simulink model "EulerPIDJoint_Copy"  (Simulink 7.6)
settings: Solver=ode3  StartTime=0.0  StopTime=8  FixedStep=Ts  RelTol=1e-3
InitFcn:
  | eval('Config');
  | eval('RobotCtlCfg');
values from neighbouring files (symbols this model uses):
  a2 = 0    [Config.m]    (also in CtrPlatformCfg.m)
  a3 = 0    [Config.m]    (also in CtrPlatformCfg.m)
  a4 = 0    [Config.m]    (also in CtrPlatformCfg.m)
  a5 = 90    [Config.m]    (also in CtrPlatformCfg.m)
  a6 = 0    [Config.m]    (also in CtrPlatformCfg.m)
  Cen_EU = Cen    [DynEulerTest.m]
  DH_EU = [266     300     0       0       1016     0      174 ... (first row only)    [DynEulerTest.m]
  freq = tvel/radius    (= 1)    [Config.m]    (also in CtrPlatformCfg.m)
  Ft_EU = [0;0;0;0;0;0]    [DynEulerTest.m]
  Gravity = 9.8    [Config.m]    (also in CtrPlatformCfg.m)
  Ie_EU = [Ie1;Ie2;Ie3;Ie4;Ie5;Ie6]    [DynEulerTest.m]
  in1 = [5.2954 -0.2565 -0.6366;-0.2565 4.7000 0.2830;-0.6366 0.2829 5.8635]    [Config.m]    (also in CtrPlatformCfg.m; DynEulerTest.m; EfDynCAD.m = [0.54  -0.01 0.23)
  in2 = [5.8840 0.0072 0.0135;0.0072 6.0178 -0.1907;0.0135 -0.1907 0.3374]    [Config.m]    (also in CtrPlatformCfg.m; DynEulerTest.m; EfDynCAD.m = (R_x*R_z)*in2*(R_x*R_z)')
  in3 = [1.8201 -0.2274 -0.3112;-0.2274 2.2537 -0.1441;-0.3112 -0.1441 1.9485]    [Config.m]    (also in CtrPlatformCfg.m; DynEulerTest.m; EfDynCAD.m = (R_x*R_z)*in3*(R_x*R_z)')
  in4 = [0.0607 -0.0922 0;-0.0922 1.4493 0;0 0 1.4620]    [Config.m]    (also in CtrPlatformCfg.m; DynEulerTest.m = [0.0607 -0.0922 0;-0.0922 1.4493 0;0 0,1.4620]; EfDynCAD.m = (R_y*Rz)*in4*(R_y*Rz)')
  in5 = [0.0191 0.0032 0;0.0032 0.0228 0;0 0 0.0291]    [Config.m]    (also in CtrPlatformCfg.m; DynEulerTest.m; EfDynCAD.m = (R_x*R_y)*in5*(R_x*R_y)')
  in6 = [0.0012 0 0;0 0.0007 0;0 0 0.0007]    [Config.m]    (also in CtrPlatformCfg.m; DynEulerTest.m; EfDynCAD.m = (R_y*Rz)*in6*(R_y*Rz)')
  init_Endx = gd_init(1,4)    [Config.m]    (also in CtrPlatformCfg.m)
  init_Endy = gd_init(2,4)    [Config.m]    (also in CtrPlatformCfg.m)
  init_Endz = gd_init(3,4)    [Config.m]    (also in CtrPlatformCfg.m)
  init_Rot = gd_init(1:3,1:3)    [Config.m]    (also in CtrPlatformCfg.m)
  L = [l1 l2 l3 l4 l5 l6 l7 l8 l9]    [Config.m]    (also in CtrPlatformCfg.m)
  ma1 = 170.31    [Config.m]    (also in CtrPlatformCfg.m; DynEulerTest.m; EfDynCAD.m = 77.75)
  ma2 = 63.74    [Config.m]    (also in CtrPlatformCfg.m; DynEulerTest.m; EfDynCAD.m = 32.31)
  ma3 = 98.98    [Config.m]    (also in CtrPlatformCfg.m; DynEulerTest.m; EfDynCAD.m = 18.61)
  ma4 = 24.46    [Config.m]    (also in CtrPlatformCfg.m; DynEulerTest.m; EfDynCAD.m = 15.65)
  ma5 = 5.24    [Config.m]    (also in CtrPlatformCfg.m; DynEulerTest.m; EfDynCAD.m = 3.32)
  ma6 = 0.6    [Config.m]    (also in CtrPlatformCfg.m; DynEulerTest.m; EfDynCAD.m)
  Ma_EU = Ma    [DynEulerTest.m]
  Rad2Line = Gear*EncRes/(2*pi)    [Config.m]    (also in CtrPlatformCfg.m)
  Ts = 1/FrHz    (= 0.00025)    [Config.m]    (also in CtrPlatformCfg.m)
  tvel = 120    [Config.m]    (also in CtrPlatformCfg.m)
undefined symbols (not defined in the file or in its folder): a1, DiscIntNeverNeededParam, jointAugKp, jointAugKv, PRBSGain, PRBSOffset, PRBSTimeLength, PulseFrq, PulseGain, RobotAxis, SineFrq, SineGain, V2T
libraries: simulink x58, mblibv1 x41, powerlib_extras x7
(part 3 of 5)

== system EulerPIDJoint_Copy/Display/GeneralForceDisplay/Jnt4 ==
  Enc : Inport
  Ref : Inport  Port=2
  Demux1 : Demux  Outputs=2
  Demux3 : Demux  Outputs=6
  Display : Subsystem
  Mux : Mux  Inputs=3
  Mux1 : Mux  Inputs=3
  Mux2 : Mux  Inputs=2
  Mux3 : Mux  Inputs=2
  Sign{1,3..4,6} (4 alike) : Gain
  Sign2 : Gain  Gain=-1
  Sign5 : Gain  Gain=-1
  wires:
  Mux3/1 -> Display/2(Ref_GeneralForce4)
  Mux2/1 -> Display/1(GeneralForce4)
  Sign5/1 -> Mux1/2
  Sign2/1 -> Mux/2
  Demux3/6 -> Sign6/1
  Demux3/5 -> Sign5/1
  Demux3/4 -> Sign4/1
  Demux3/3 -> Sign3/1
  Demux3/2 -> Sign2/1
  Demux3/1 -> Sign1/1
  Mux1/1 -> Mux3/2
  Mux/1 -> Mux3/1
  Ref/1 -> Demux3/1
  Enc/1 -> Demux1/1
  Sign1/1 -> Mux/3
  Sign3/1 -> Mux/1
  Sign4/1 -> Mux1/3
  Sign6/1 -> Mux1/1
  Demux1/1 -> Mux2/1
  Demux1/2 -> Mux2/2

== system EulerPIDJoint_Copy/Display/GeneralForceDisplay/Jnt5 ==
  Enc : Inport
  Ref : Inport  Port=2
  Demux1 : Demux  Outputs=2
  Demux3 : Demux  Outputs=6
  Display : Subsystem
  Mux : Mux  Inputs=3
  Mux1 : Mux  Inputs=3
  Mux2 : Mux  Inputs=2
  Mux3 : Mux  Inputs=2
  Sign{1,3..4,6} (4 alike) : Gain  Gain=-1
  Sign2 : Gain
  Sign5 : Gain
  wires:
  Enc/1 -> Demux1/1
  Ref/1 -> Demux3/1
  Mux/1 -> Mux3/1
  Mux1/1 -> Mux3/2
  Demux3/1 -> Sign1/1
  Demux3/2 -> Sign2/1
  Demux3/3 -> Sign3/1
  Demux3/4 -> Sign4/1
  Demux3/5 -> Sign5/1
  Demux3/6 -> Sign6/1
  Mux2/1 -> Display/1(GeneralForce5)
  Mux3/1 -> Display/2(Ref_GeneralForce5)
  Sign1/1 -> Mux/2
  Sign2/1 -> Mux/3
  Sign3/1 -> Mux/1
  Sign4/1 -> Mux1/2
  Sign5/1 -> Mux1/3
  Sign6/1 -> Mux1/1
  Demux1/1 -> Mux2/1
  Demux1/2 -> Mux2/2

== system EulerPIDJoint_Copy/Display/GeneralForceDisplay/Jnt6 ==
  Enc : Inport
  Ref : Inport  Port=2
  Demux1 : Demux  Outputs=2
  Demux3 : Demux  Outputs=6
  Display : Subsystem
  Mux : Mux  Inputs=3
  Mux1 : Mux  Inputs=3
  Mux2 : Mux  Inputs=2
  Mux3 : Mux  Inputs=2
  Sign{1,3..4,6} (4 alike) : Gain
  Sign2 : Gain  Gain=-1
  Sign5 : Gain  Gain=-1
  wires:
  Mux3/1 -> Display/2(Ref_GeneralForce6)
  Mux2/1 -> Display/1(GeneralForce6)
  Sign5/1 -> Mux1/2
  Sign2/1 -> Mux/2
  Demux3/6 -> Sign6/1
  Demux3/5 -> Sign5/1
  Demux3/4 -> Sign4/1
  Demux3/3 -> Sign3/1
  Demux3/2 -> Sign2/1
  Demux3/1 -> Sign1/1
  Mux1/1 -> Mux3/2
  Mux/1 -> Mux3/1
  Ref/1 -> Demux3/1
  Enc/1 -> Demux1/1
  Sign1/1 -> Mux/3
  Sign3/1 -> Mux/1
  Sign6/1 -> Mux1/1
  Sign4/1 -> Mux1/3
  Demux1/1 -> Mux2/1
  Demux1/2 -> Mux2/2

== system EulerPIDJoint_Copy/Display/GeneralVelDisplay/Jnt1 ==
  Enc : Inport
  Ref : Inport  Port=2
  Demux1 : Demux  Outputs=2
  Demux3 : Demux  Outputs=6
  Display : Subsystem
  Mux : Mux  Inputs=3
  Mux1 : Mux  Inputs=3
  Mux2 : Mux  Inputs=2
  Mux3 : Mux  Inputs=2
  Sign{1..6} (6 alike) : Gain
  wires:
  Enc/1 -> Demux1/1
  Ref/1 -> Demux3/1
  Mux/1 -> Mux3/1
  Mux1/1 -> Mux3/2
  Demux3/1 -> Sign1/1
  Demux3/2 -> Sign2/1
  Demux3/3 -> Sign3/1
  Demux3/4 -> Sign4/1
  Demux3/5 -> Sign5/1
  Demux3/6 -> Sign6/1
  Sign1/1 -> Mux/1
  Sign2/1 -> Mux/2
  Sign3/1 -> Mux/3
  Sign4/1 -> Mux1/1
  Sign5/1 -> Mux1/2
  Sign6/1 -> Mux1/3
  Demux1/1 -> Mux2/1
  Demux1/2 -> Mux2/2
  Mux2/1 -> Display/1(GeneralVel1)
  Mux3/1 -> Display/2(Ref_GeneralVel1)

== system EulerPIDJoint_Copy/Display/GeneralVelDisplay/Jnt2 ==
  Enc : Inport
  Ref : Inport  Port=2
  Demux1 : Demux  Outputs=2
  Demux3 : Demux  Outputs=6
  Display : Subsystem
  Mux : Mux  Inputs=3
  Mux1 : Mux  Inputs=3
  Mux2 : Mux  Inputs=2
  Mux3 : Mux  Inputs=2
  Sign{1..2,4..5} (4 alike) : Gain
  Sign3 : Gain  Gain=-1
  Sign6 : Gain  Gain=-1
  wires:
  Mux3/1 -> Display/2(Ref_GeneralVel2)
  Mux2/1 -> Display/1(GeneralVel2)
  Demux1/2 -> Mux2/2
  Demux1/1 -> Mux2/1
  Sign4/1 -> Mux1/1
  Sign1/1 -> Mux/1
  Demux3/6 -> Sign6/1
  Demux3/5 -> Sign5/1
  Demux3/4 -> Sign4/1
  Demux3/3 -> Sign3/1
  Demux3/2 -> Sign2/1
  Demux3/1 -> Sign1/1
  Mux1/1 -> Mux3/2
  Mux/1 -> Mux3/1
  Ref/1 -> Demux3/1
  Enc/1 -> Demux1/1
  Sign3/1 -> Mux/2
  Sign2/1 -> Mux/3
  Sign6/1 -> Mux1/2
  Sign5/1 -> Mux1/3

== system EulerPIDJoint_Copy/Display/GeneralVelDisplay/Jnt3 ==
  Enc : Inport
  Ref : Inport  Port=2
  Demux1 : Demux  Outputs=2
  Demux3 : Demux  Outputs=6
  Display : Subsystem
  Mux : Mux  Inputs=3
  Mux1 : Mux  Inputs=3
  Mux2 : Mux  Inputs=2
  Mux3 : Mux  Inputs=2
  Sign{1..6} (6 alike) : Gain
  wires:
  Enc/1 -> Demux1/1
  Ref/1 -> Demux3/1
  Mux/1 -> Mux3/1
  Mux1/1 -> Mux3/2
  Demux3/1 -> Sign1/1
  Demux3/2 -> Sign2/1
  Demux3/3 -> Sign3/1
  Demux3/4 -> Sign4/1
  Demux3/5 -> Sign5/1
  Demux3/6 -> Sign6/1
  Demux1/1 -> Mux2/1
  Demux1/2 -> Mux2/2
  Mux2/1 -> Display/1(GeneralVel3)
  Mux3/1 -> Display/2(Ref_GeneralVel3)
  Sign1/1 -> Mux/2
  Sign2/1 -> Mux/3
  Sign3/1 -> Mux/1
  Sign4/1 -> Mux1/2
  Sign6/1 -> Mux1/1
  Sign5/1 -> Mux1/3

== system EulerPIDJoint_Copy/Display/GeneralVelDisplay/Jnt4 ==
  Enc : Inport
  Ref : Inport  Port=2
  Demux1 : Demux  Outputs=2
  Demux3 : Demux  Outputs=6
  Display : Subsystem
  Mux : Mux  Inputs=3
  Mux1 : Mux  Inputs=3
  Mux2 : Mux  Inputs=2
  Mux3 : Mux  Inputs=2
  Sign{1,3..4,6} (4 alike) : Gain
  Sign2 : Gain  Gain=-1
  Sign5 : Gain  Gain=-1
  wires:
  Mux3/1 -> Display/2(Ref_GeneralVel4)
  Mux2/1 -> Display/1(GeneralVel4)
  Sign5/1 -> Mux1/2
  Sign2/1 -> Mux/2
  Demux3/6 -> Sign6/1
  Demux3/5 -> Sign5/1
  Demux3/4 -> Sign4/1
  Demux3/3 -> Sign3/1
  Demux3/2 -> Sign2/1
  Demux3/1 -> Sign1/1
  Mux1/1 -> Mux3/2
  Mux/1 -> Mux3/1
  Ref/1 -> Demux3/1
  Enc/1 -> Demux1/1
  Sign1/1 -> Mux/3
  Sign3/1 -> Mux/1
  Sign4/1 -> Mux1/3
  Sign6/1 -> Mux1/1
  Demux1/1 -> Mux2/1
  Demux1/2 -> Mux2/2

== system EulerPIDJoint_Copy/Display/GeneralVelDisplay/Jnt5 ==
  Enc : Inport
  Ref : Inport  Port=2
  Demux1 : Demux  Outputs=2
  Demux3 : Demux  Outputs=6
  Display : Subsystem
  Mux : Mux  Inputs=3
  Mux1 : Mux  Inputs=3
  Mux2 : Mux  Inputs=2
  Mux3 : Mux  Inputs=2
  Sign{1,3..4,6} (4 alike) : Gain  Gain=-1
  Sign2 : Gain
  Sign5 : Gain
  wires:
  Enc/1 -> Demux1/1
  Ref/1 -> Demux3/1
  Mux/1 -> Mux3/1
  Mux1/1 -> Mux3/2
  Demux3/1 -> Sign1/1
  Demux3/2 -> Sign2/1
  Demux3/3 -> Sign3/1
  Demux3/4 -> Sign4/1
  Demux3/5 -> Sign5/1
  Demux3/6 -> Sign6/1
  Mux2/1 -> Display/1(GeneralVel5)
  Mux3/1 -> Display/2(Ref_GeneralVel5)
  Sign1/1 -> Mux/2
  Sign2/1 -> Mux/3
  Sign3/1 -> Mux/1
  Sign4/1 -> Mux1/2
  Sign5/1 -> Mux1/3
  Sign6/1 -> Mux1/1
  Demux1/1 -> Mux2/1
  Demux1/2 -> Mux2/2

== system EulerPIDJoint_Copy/Display/GeneralVelDisplay/Jnt6 ==
  Enc : Inport
  Ref : Inport  Port=2
  Demux1 : Demux  Outputs=2
  Demux3 : Demux  Outputs=6
  Display : Subsystem
  Mux : Mux  Inputs=3
  Mux1 : Mux  Inputs=3
  Mux2 : Mux  Inputs=2
  Mux3 : Mux  Inputs=2
  Sign{1,3..4,6} (4 alike) : Gain
  Sign2 : Gain  Gain=-1
  Sign5 : Gain  Gain=-1
  wires:
  Mux3/1 -> Display/2(Ref_GeneralVel6)
  Mux2/1 -> Display/1(GeneralVel6)
  Sign5/1 -> Mux1/2
  Sign2/1 -> Mux/2
  Demux3/6 -> Sign6/1
  Demux3/5 -> Sign5/1
  Demux3/4 -> Sign4/1
  Demux3/3 -> Sign3/1
  Demux3/2 -> Sign2/1
  Demux3/1 -> Sign1/1
  Mux1/1 -> Mux3/2
  Mux/1 -> Mux3/1
  Ref/1 -> Demux3/1
  Enc/1 -> Demux1/1
  Sign1/1 -> Mux/3
  Sign3/1 -> Mux/1
  Sign6/1 -> Mux1/1
  Sign4/1 -> Mux1/3
  Demux1/1 -> Mux2/1
  Demux1/2 -> Mux2/2

== system EulerPIDJoint_Copy/Display/JntVelAccDisplay/Joint1 ==
  JVA1 : Inport
  Ref_JVA1 : Inport  Port=2
  Acceleration : Scope
      settings: SaveName=ScopeData2
  Angle : Scope
      settings: TimeRange=10  YMin=-3e-017  YMax=4e-017
  Demux : Demux  Outputs=3
  Demux1 : Demux  Outputs=3
  "Encoder " : ToWorkspace  VariableName=EncJVAJ1  SampleTime=-1  SaveFormat=Structure
  Err1 : Scope
      settings: SaveName=ScopeData6
  Err2 : Scope
      settings: SaveName=ScopeData7
  Err3 : Scope
      settings: SaveName=ScopeData8
  Mux : Mux  Inputs=2
  Mux1 : Mux  Inputs=2
  Mux2 : Mux  Inputs=2
  "Ref " : ToWorkspace  VariableName=RefJVAJ1  SampleTime=-1  SaveFormat=Structure
  Sum : Sum  Inputs=+|-
  Sum1 : Sum  Inputs=+|-
  Sum2 : Sum  Inputs=+|-
  "Velocity " : Scope
  wires:
  Ref_JVA1/1 -> "Ref "/1, Demux1/1
  JVA1/1 -> "Encoder "/1, Demux/1
  Sum2/1 -> Err3/1
  Sum1/1 -> Err2/1
  Sum/1 -> Err1/1
  Demux/1 -> Sum/1, Mux/1
  Demux1/1 -> Sum/2, Mux/2
  Demux/2 -> Sum1/1, Mux1/1
  Demux1/2 -> Sum1/2, Mux1/2
  Demux/3 -> Sum2/1, Mux2/1
  Demux1/3 -> Sum2/2, Mux2/2
  Mux/1 -> Angle/1
  Mux1/1 -> "Velocity "/1
  Mux2/1 -> Acceleration/1

== system EulerPIDJoint_Copy/Display/JntVelAccDisplay/Joint2 ==
  JVA2 : Inport
  Ref_JVA2 : Inport  Port=2
  Acceleration : Scope
      settings: SaveName=ScopeData2
  Angle : Scope
      settings: TimeRange=10  YMin=-3e-017  YMax=4e-017
  Demux : Demux  Outputs=3
  Demux1 : Demux  Outputs=3
  "Encoder " : ToWorkspace  VariableName=EncJVAJ2  SampleTime=-1  SaveFormat=Structure
  Err1 : Scope
      settings: SaveName=ScopeData6
  Err2 : Scope
      settings: SaveName=ScopeData7
  Err3 : Scope
      settings: SaveName=ScopeData8
  Mux : Mux  Inputs=2
  Mux1 : Mux  Inputs=2
  Mux2 : Mux  Inputs=2
  "Ref " : ToWorkspace  VariableName=RefJVAJ2  SampleTime=-1  SaveFormat=Structure
  Sum : Sum  Inputs=+|-
  Sum1 : Sum  Inputs=+|-
  Sum2 : Sum  Inputs=+|-
  "Velocity " : Scope
  wires:
  Mux2/1 -> Acceleration/1
  Mux1/1 -> "Velocity "/1
  Mux/1 -> Angle/1
  Demux1/3 -> Mux2/2, Sum2/2
  Demux/3 -> Mux2/1, Sum2/1
  Demux1/2 -> Mux1/2, Sum1/2
  Demux/2 -> Mux1/1, Sum1/1
  Demux1/1 -> Mux/2, Sum/2
  Demux/1 -> Mux/1, Sum/1
  Sum/1 -> Err1/1
  Sum1/1 -> Err2/1
  Sum2/1 -> Err3/1
  JVA2/1 -> Demux/1, "Encoder "/1
  Ref_JVA2/1 -> Demux1/1, "Ref "/1

== system EulerPIDJoint_Copy/Display/JntVelAccDisplay/Joint3 ==
  JVA3 : Inport
  Ref_JVA3 : Inport  Port=2
  Acceleration : Scope
      settings: SaveName=ScopeData2
  Angle : Scope
      settings: TimeRange=10  YMin=-3e-017  YMax=4e-017
  Demux : Demux  Outputs=3
  Demux1 : Demux  Outputs=3
  "Encoder " : ToWorkspace  VariableName=EncJVAJ3  SampleTime=-1  SaveFormat=Structure
  Err1 : Scope
      settings: SaveName=ScopeData6
  Err2 : Scope
      settings: SaveName=ScopeData7
  Err3 : Scope
      settings: SaveName=ScopeData8
  Mux : Mux  Inputs=2
  Mux1 : Mux  Inputs=2
  Mux2 : Mux  Inputs=2
  "Ref " : ToWorkspace  VariableName=RefJVAJ3  SampleTime=-1  SaveFormat=Structure
  Sum : Sum  Inputs=+|-
  Sum1 : Sum  Inputs=+|-
  Sum2 : Sum  Inputs=+|-
  "Velocity " : Scope
  wires:
  Ref_JVA3/1 -> "Ref "/1, Demux1/1
  JVA3/1 -> "Encoder "/1, Demux/1
  Sum2/1 -> Err3/1
  Sum1/1 -> Err2/1
  Sum/1 -> Err1/1
  Demux/1 -> Sum/1, Mux/1
  Demux1/1 -> Sum/2, Mux/2
  Demux/2 -> Sum1/1, Mux1/1
  Demux1/2 -> Sum1/2, Mux1/2
  Demux/3 -> Sum2/1, Mux2/1
  Demux1/3 -> Sum2/2, Mux2/2
  Mux/1 -> Angle/1
  Mux1/1 -> "Velocity "/1
  Mux2/1 -> Acceleration/1

== system EulerPIDJoint_Copy/Display/JntVelAccDisplay/Joint4 ==
  JVA4 : Inport
  Ref_JVA4 : Inport  Port=2
  Acceleration : Scope
      settings: SaveName=ScopeData2
  Angle : Scope
      settings: TimeRange=10  YMin=-3e-017  YMax=4e-017
  Demux : Demux  Outputs=3
  Demux1 : Demux  Outputs=3
  "Encoder " : ToWorkspace  VariableName=EncJVAJ4  SampleTime=-1  SaveFormat=Structure
  Err1 : Scope
      settings: SaveName=ScopeData6
  Err2 : Scope
      settings: SaveName=ScopeData7
  Err3 : Scope
      settings: SaveName=ScopeData8
  Mux : Mux  Inputs=2
  Mux1 : Mux  Inputs=2
  Mux2 : Mux  Inputs=2
  "Ref " : ToWorkspace  VariableName=RefJVAJ4  SampleTime=-1  SaveFormat=Structure
  Sum : Sum  Inputs=+|-
  Sum1 : Sum  Inputs=+|-
  Sum2 : Sum  Inputs=+|-
  "Velocity " : Scope
  wires:
  Mux2/1 -> Acceleration/1
  Mux1/1 -> "Velocity "/1
  Mux/1 -> Angle/1
  Demux1/3 -> Mux2/2, Sum2/2
  Demux/3 -> Mux2/1, Sum2/1
  Demux1/2 -> Mux1/2, Sum1/2
  Demux/2 -> Mux1/1, Sum1/1
  Demux1/1 -> Mux/2, Sum/2
  Demux/1 -> Mux/1, Sum/1
  Sum/1 -> Err1/1
  Sum1/1 -> Err2/1
  Sum2/1 -> Err3/1
  JVA4/1 -> Demux/1, "Encoder "/1
  Ref_JVA4/1 -> Demux1/1, "Ref "/1

== system EulerPIDJoint_Copy/Display/JntVelAccDisplay/Joint5 ==
  JVA5 : Inport
  Ref_JVA5 : Inport  Port=2
  Acceleration : Scope
      settings: SaveName=ScopeData2
  Angle : Scope
      settings: TimeRange=10  YMin=-3e-017  YMax=4e-017
  Demux : Demux  Outputs=3
  Demux1 : Demux  Outputs=3
  "Encoder " : ToWorkspace  VariableName=EncJVAJ5  SampleTime=-1  SaveFormat=Structure
  Err1 : Scope
      settings: SaveName=ScopeData6
  Err2 : Scope
      settings: SaveName=ScopeData7
  Err3 : Scope
      settings: SaveName=ScopeData8
  Mux : Mux  Inputs=2
  Mux1 : Mux  Inputs=2
  Mux2 : Mux  Inputs=2
  "Ref " : ToWorkspace  VariableName=RefJVAJ5  SampleTime=-1  SaveFormat=Structure
  Sum : Sum  Inputs=+|-
  Sum1 : Sum  Inputs=+|-
  Sum2 : Sum  Inputs=+|-
  "Velocity " : Scope
  wires:
  Ref_JVA5/1 -> "Ref "/1, Demux1/1
  JVA5/1 -> "Encoder "/1, Demux/1
  Sum2/1 -> Err3/1
  Sum1/1 -> Err2/1
  Sum/1 -> Err1/1
  Demux/1 -> Sum/1, Mux/1
  Demux1/1 -> Sum/2, Mux/2
  Demux/2 -> Sum1/1, Mux1/1
  Demux1/2 -> Sum1/2, Mux1/2
  Demux/3 -> Sum2/1, Mux2/1
  Demux1/3 -> Sum2/2, Mux2/2
  Mux/1 -> Angle/1
  Mux1/1 -> "Velocity "/1
  Mux2/1 -> Acceleration/1

== system EulerPIDJoint_Copy/Display/JntVelAccDisplay/Joint6 ==
  JVA6 : Inport
  Ref_JVA6 : Inport  Port=2
  Acceleration : Scope
      settings: SaveName=ScopeData2
  Angle : Scope
      settings: TimeRange=10  YMin=-3e-017  YMax=4e-017
  Demux : Demux  Outputs=3
  Demux1 : Demux  Outputs=3
  "Encoder " : ToWorkspace  VariableName=EncJVAJ6  SampleTime=-1  SaveFormat=Structure
  Err1 : Scope
      settings: SaveName=ScopeData6
  Err2 : Scope
      settings: SaveName=ScopeData7
  Err3 : Scope
      settings: SaveName=ScopeData8
  Mux : Mux  Inputs=2
  Mux1 : Mux  Inputs=2
  Mux2 : Mux  Inputs=2
  "Ref " : ToWorkspace  VariableName=RefJVAJ6  SampleTime=-1  SaveFormat=Structure
  Sum : Sum  Inputs=+|-
  Sum1 : Sum  Inputs=+|-
  Sum2 : Sum  Inputs=+|-
  "Velocity " : Scope
  wires:
  Mux2/1 -> Acceleration/1
  Mux1/1 -> "Velocity "/1
  Mux/1 -> Angle/1
  Demux1/3 -> Mux2/2, Sum2/2
  Demux/3 -> Mux2/1, Sum2/1
  Demux1/2 -> Mux1/2, Sum1/2
  Demux/2 -> Mux1/1, Sum1/1
  Demux1/1 -> Mux/2, Sum/2
  Demux/1 -> Mux/1, Sum/1
  Sum/1 -> Err1/1
  Sum1/1 -> Err2/1
  Sum2/1 -> Err3/1
  JVA6/1 -> Demux/1, "Encoder "/1
  Ref_JVA6/1 -> Demux1/1, "Ref "/1

== system EulerPIDJoint_Copy/Trajectory Generator/Circle in Descartes Space/EndVelocity ==
  Constant : Constant  Value=-1  SampleTime=Ts
  End_Vx : Sin  Amplitude=-tvel  Frequency=freq  SampleTime=Ts
  End_Vy : Sin  Frequency=freq  Phase=pi/2  SampleTime=Ts
  End_Vz : Constant  Value=0  SampleTime=Ts
  Gain : Gain  Gain=tvel
  Integer Delay : simulink/Discrete/Integer Delay  NumDelays=1/Ts  vinit=0.0  samptime=-1
  Integer Delay1 : simulink/Discrete/Integer Delay  NumDelays=1/Ts  vinit=0.0  samptime=-1
  Ramp : simulink/Sources/Ramp  SystemSampleTime=-1  slope=1  start=0  X0=0
  Ramp1 : simulink/Sources/Ramp  SystemSampleTime=-1  slope=-1  start=1  X0=0
  Sum : Sum  Inputs=|++
  Sum1 : Sum  Inputs=++|  SampleTime=Ts
  Sum2 : Sum  Inputs=++|
  EndVx : Outport
  EndVy : Outport  Port=2
  EndVz : Outport  Port=3
  wires:
  End_Vy/1 -> Sum2/1
  Ramp/1 -> Sum/1
  Ramp1/1 -> Sum/2
  Integer Delay1/1 -> Sum1/1
  Sum2/1 -> Integer Delay1/1
  Constant/1 -> Sum2/2
  Sum/1 -> Sum1/2
  Sum1/1 -> Gain/1
  End_Vx/1 -> Integer Delay/1
  End_Vz/1 -> EndVx/1
  Gain/1 -> EndVy/1
  Integer Delay/1 -> EndVz/1

== system EulerPIDJoint_Copy/Trajectory Generator/Circle in Descartes Space/Re-group  ==
  JJVVAA : Inport
  Demux2 : Demux  Outputs=18
  Mux{,1..2,4..6} (6 alike) : Mux  Inputs=3
  Mux3 : Mux  Inputs=6
  JVAJVA : Outport
  wires:
  JJVVAA/1 -> Demux2/1
  Mux3/1 -> JVAJVA/1
  Mux/1 -> Mux3/1
  Mux1/1 -> Mux3/2
  Mux2/1 -> Mux3/3
  Mux4/1 -> Mux3/4
  Mux5/1 -> Mux3/5
  Mux6/1 -> Mux3/6
  Demux2/1 -> Mux/1
  Demux2/2 -> Mux1/1
  Demux2/3 -> Mux2/1
  Demux2/4 -> Mux4/1
  Demux2/5 -> Mux5/1
  Demux2/6 -> Mux6/1
  Demux2/7 -> Mux/2
  Demux2/8 -> Mux1/2
  Demux2/9 -> Mux2/2
  Demux2/10 -> Mux4/2
  Demux2/11 -> Mux5/2
  Demux2/12 -> Mux6/2
  Demux2/13 -> Mux/3
  Demux2/14 -> Mux1/3
  Demux2/15 -> Mux2/3
  Demux2/16 -> Mux4/3
  Demux2/17 -> Mux5/3
  Demux2/18 -> Mux6/3

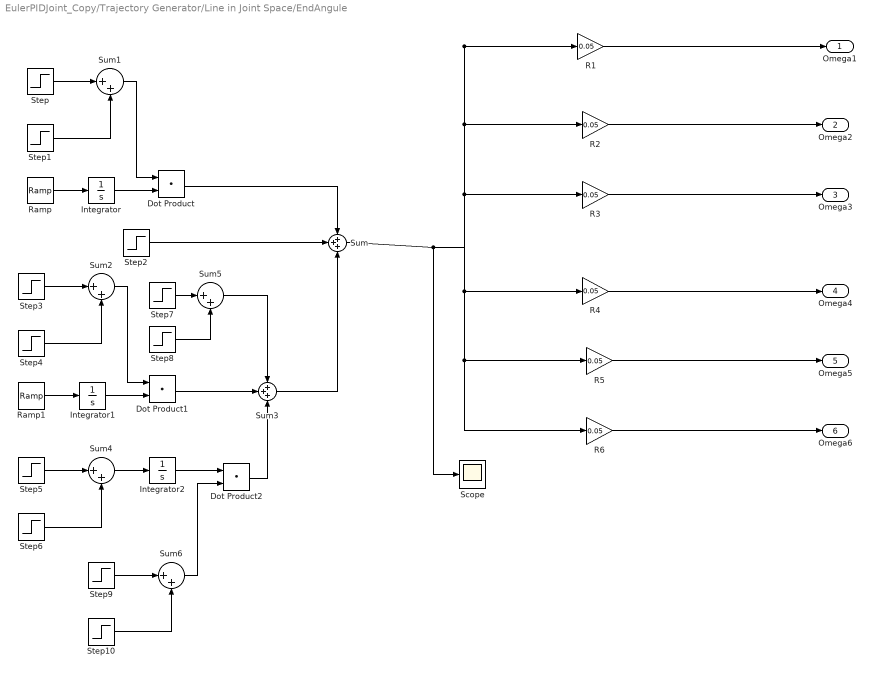
== system EulerPIDJoint_Copy/Trajectory Generator/Line in Joint Space/EndAngule ==
  Dot Product : DotProduct  InputSameDT=on  OutDataTypeStr=Inherit: Inherit via internal rule
  Dot Product1 : DotProduct  InputSameDT=on  OutDataTypeStr=Inherit: Inherit via internal rule
  Dot Product2 : DotProduct  InputSameDT=on  OutDataTypeStr=Inherit: Inherit via internal rule
  Integrator : Integrator
  Integrator1 : Integrator
  Integrator2 : Integrator
  R{1..6} (6 alike) : Gain  Gain=0.05
  Ramp : simulink/Sources/Ramp  SystemSampleTime=-1  slope=1  start=0  X0=0
  Ramp1 : simulink/Sources/Ramp  SystemSampleTime=-1  slope=-1  start=0  X0=0
  Scope : Scope
      settings: SaveName=ScopeData21
  Step : Step  After=-1  SampleTime=0
  Step1 : Step  Time=0  SampleTime=0
  Step10 : Step  SampleTime=0
  Step2 : Step  Time=2  SampleTime=0
  Step3 : Step  Time=2  After=-1  SampleTime=0
  Step4 : Step  SampleTime=0
  Step5 : Step  Time=2  After=-2  SampleTime=0
  Step6 : Step  After=2  SampleTime=0
  Step7 : Step  Time=2  After=-1  SampleTime=0
  Step8 : Step  SampleTime=0
  Step9 : Step  Time=2  After=-1  SampleTime=0
  Sum : Sum  Inputs=+++
  Sum{1..2,4..6} (5 alike) : Sum  Inputs=|++
  Sum3 : Sum  Inputs=+++
  Omega1 : Outport
  Omega2 : Outport  Port=2
  Omega3 : Outport  Port=3
  Omega4 : Outport  Port=4
  Omega5 : Outport  Port=5
  Omega6 : Outport  Port=6
  wires:
  R4/1 -> Omega4/1
  R6/1 -> Omega6/1
  R5/1 -> Omega5/1
  R3/1 -> Omega3/1
  R2/1 -> Omega2/1
  Ramp/1 -> Integrator/1
  R1/1 -> Omega1/1
  Sum/1 -> R1/1, R2/1, R3/1, R4/1, R5/1, R6/1, Scope/1
  Integrator/1 -> Dot Product/2
  Step/1 -> Sum1/1
  Sum1/1 -> Dot Product/1
  Step1/1 -> Sum1/2
  Dot Product/1 -> Sum/1
  Step2/1 -> Sum/2
  Ramp1/1 -> Integrator1/1
  Integrator1/1 -> Dot Product1/2
  Step3/1 -> Sum2/1
  Sum2/1 -> Dot Product1/1
  Step4/1 -> Sum2/2
  Sum3/1 -> Sum/3
  Step5/1 -> Sum4/1
  Step6/1 -> Sum4/2
  Sum4/1 -> Integrator2/1
  Dot Product1/1 -> Sum3/2
  Step7/1 -> Sum5/1
  Step8/1 -> Sum5/2
  Sum5/1 -> Sum3/1
  Step9/1 -> Sum6/1
  Step10/1 -> Sum6/2
  Integrator2/1 -> Dot Product2/1
  Sum6/1 -> Dot Product2/2
  Dot Product2/1 -> Sum3/3

== system EulerPIDJoint_Copy/Trajectory Generator/Line in Joint Space/Re-group  ==
  JJVVAA : Inport
  Demux2 : Demux  Outputs=18
  Mux{,1..2,4..6} (6 alike) : Mux  Inputs=3
  Mux3 : Mux  Inputs=6
  JVAJVA : Outport
  wires:
  JJVVAA/1 -> Demux2/1
  Mux3/1 -> JVAJVA/1
  Mux/1 -> Mux3/1
  Mux1/1 -> Mux3/2
  Mux2/1 -> Mux3/3
  Mux4/1 -> Mux3/4
  Mux5/1 -> Mux3/5
  Mux6/1 -> Mux3/6
  Demux2/1 -> Mux/1
  Demux2/2 -> Mux1/1
  Demux2/3 -> Mux2/1
  Demux2/4 -> Mux4/1
  Demux2/5 -> Mux5/1
  Demux2/6 -> Mux6/1
  Demux2/7 -> Mux/2
  Demux2/8 -> Mux1/2
  Demux2/9 -> Mux2/2
  Demux2/10 -> Mux4/2
  Demux2/11 -> Mux5/2
  Demux2/12 -> Mux6/2
  Demux2/13 -> Mux/3
  Demux2/14 -> Mux1/3
  Demux2/15 -> Mux2/3
  Demux2/16 -> Mux4/3
  Demux2/17 -> Mux5/3
  Demux2/18 -> Mux6/3

== system EulerPIDJoint_Copy/Trajectory Generator/Still/EndVelocity ==
  Constant : Constant  Value=0
  Constant1 : Constant  Value=0
  Constant2 : Constant  Value=0
  EndVx : Outport
  EndVy : Outport  Port=2
  EndVz : Outport  Port=3
  wires:
  Constant/1 -> EndVx/1
  Constant1/1 -> EndVy/1
  Constant2/1 -> EndVz/1

== system EulerPIDJoint_Copy/Trajectory Generator/Still/Re-group  ==
  JJVVAA : Inport
  Demux2 : Demux  Outputs=18
  Mux{,1..2,4..6} (6 alike) : Mux  Inputs=3
  Mux3 : Mux  Inputs=6
  JVAJVA : Outport
  wires:
  Demux2/18 -> Mux6/3
  Demux2/17 -> Mux5/3
  Demux2/16 -> Mux4/3
  Demux2/15 -> Mux2/3
  Demux2/14 -> Mux1/3
  Demux2/13 -> Mux/3
  Demux2/12 -> Mux6/2
  Demux2/11 -> Mux5/2
  Demux2/10 -> Mux4/2
  Demux2/9 -> Mux2/2
  Demux2/8 -> Mux1/2
  Demux2/7 -> Mux/2
  Demux2/6 -> Mux6/1
  Demux2/5 -> Mux5/1
  Demux2/4 -> Mux4/1
  Demux2/3 -> Mux2/1
  Demux2/2 -> Mux1/1
  Demux2/1 -> Mux/1
  Mux6/1 -> Mux3/6
  Mux5/1 -> Mux3/5
  Mux4/1 -> Mux3/4
  Mux2/1 -> Mux3/3
  Mux1/1 -> Mux3/2
  Mux/1 -> Mux3/1
  Mux3/1 -> JVAJVA/1
  JJVVAA/1 -> Demux2/1

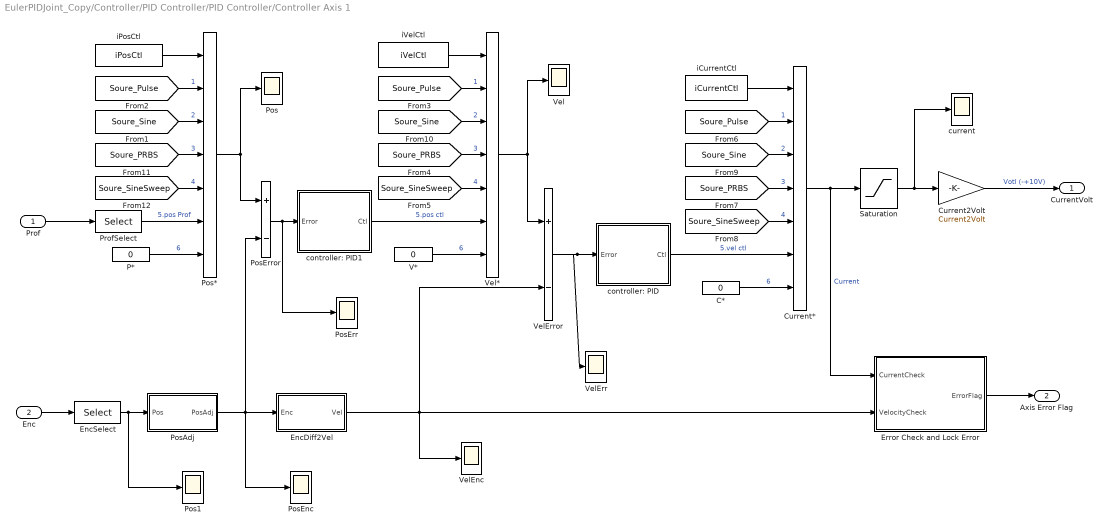
== system EulerPIDJoint_Copy/Controller/PID Controller/PID Controller/Controller Axis 1 ==
  Prof : Inport
  Enc : Inport  Port=2
  C* : Constant  Value=0  SampleTime=Ts
  Current* : MultiPortSwitch  Inputs=6  zeroidx=off
  Current2Volt : Gain  Gain=Current2Volt
  EncDiff2Vel : Subsystem
  "EncSelect " : Selector  InputPortWidth=6  IndexOptions=Index vector (dialog)  Indices=AxisNO  OutputSizes=1
  Error Check and Lock Error : Subsystem
  P* : Constant  Value=0  SampleTime=Ts
  Pos : Scope
      settings: TimeRange=1.4  YMin=-1  YMax=1  SaveName=ScopeData2
  Pos* : MultiPortSwitch  Inputs=6  zeroidx=off
  Pos1 : Scope
      settings: TimeRange=10  YMin=-1  YMax=1  SaveName=ScopeData43
  PosAdj : Subsystem
  PosEnc : Scope
      settings: TimeRange=10  YMin=-1  YMax=1  SaveName=ScopeData44
  PosErr : Scope
      settings: TimeRange=10  YMin=-1  YMax=1  SaveName=ScopeData42
  PosError : Sum  Inputs=+-
  ProfSelect : Selector  InputPortWidth=6  IndexOptions=Index vector (dialog)  Indices=AxisNO  OutputSizes=1
  Saturation : Saturate  UpperLimit=VLLimit %A  LowerLimit=-VLLimit %A  SampleTime=Ts
      settings: AttributesFormatString=%<UpperLimit>\n%<LowerLimit>
  V* : Constant  Value=0  SampleTime=Ts
  Vel : Scope
      settings: TimeRange=10  YMin=-1  YMax=1  SaveName=ScopeData5
  Vel* : MultiPortSwitch  Inputs=6  zeroidx=off
  VelEnc : Scope
      settings: TimeRange=10  YMin=-1  YMax=1  SaveName=ScopeData45
  VelErr : Scope
      settings: TimeRange=10  YMin=-1  YMax=1  SaveName=ScopeData46
  VelError : Sum  Inputs=+-
  controller: PID : Subsystem  mask{Kp=VLKp, Ki=VLKi, Kd=0, LimitSet=VLLimit, Ts=Ts}
      mask prompts: LimitSet "Limit of Int"; Ts "Sample Time"
  controller: PID1 : Subsystem  mask{Kp=PLKp, Ki=0, Kd=0, LimitSet=PLLimit, Ts=Ts}
      mask prompts: LimitSet "Limit of Int"; Ts "Sample Time"
  current : Scope
      settings: TimeRange=12  YMin=-9  YMax=9  SaveName=ScopeData3
  iCurrentCtl : Constant  Value=iCurrentCtl  SampleTime=Ts
  iPosCtl : Constant  Value=iPosCtl  SampleTime=Ts
  iVelCtl : Constant  Value=iVelCtl  SampleTime=Ts
  CurrentVolt : Outport
  Axis Error Flag : Outport  Port=2
  wires:
  Error Check and Lock Error/1(ErrorFlag) -> Axis Error Flag/1
  Saturation/1 -> current/1, Current2Volt/1
  Current*/1 -> Error Check and Lock Error/1(CurrentCheck), Saturation/1  "Current"
  PosError/1 -> controller: PID1/1(Error), PosErr/1
  iCurrentCtl/1 -> Current*/1
  iVelCtl/1 -> Vel*/1
  VelError/1 -> controller: PID/1(Error), VelErr/1
  controller: PID1/1(Ctl) -> Vel*/6  "5.pos ctl"
  PosAdj/1(PosAdj) -> EncDiff2Vel/1(Enc), PosEnc/1, PosError/2
  EncDiff2Vel/1(Vel) -> Error Check and Lock Error/2(VelocityCheck), VelEnc/1, VelError/2
  Prof/1 -> ProfSelect/1
  Enc/1 -> "EncSelect "/1
  "EncSelect "/1 -> PosAdj/1(Pos), Pos1/1
  [Soure_Pulse] -> Current*/2  "1"
  [Soure_Sine] -> Current*/3  "2"
  [Soure_PRBS] -> Current*/4  "3"
  [Soure_SineSweep] -> Current*/5  "4"
  controller: PID/1(Ctl) -> Current*/6  "5.vel ctl"
  C*/1 -> Current*/7  "6"
  [Soure_Pulse] -> Vel*/2  "1"
  [Soure_Sine] -> Vel*/3  "2"
  [Soure_PRBS] -> Vel*/4  "3"
  [Soure_SineSweep] -> Vel*/5  "4"
  V*/1 -> Vel*/7  "6"
  Vel*/1 -> Vel/1, VelError/1
  iPosCtl/1 -> Pos*/1
  ProfSelect/1 -> Pos*/6  "5.pos Prof"
  [Soure_Pulse] -> Pos*/2  "1"
  [Soure_Sine] -> Pos*/3  "2"
  [Soure_PRBS] -> Pos*/4  "3"
  [Soure_SineSweep] -> Pos*/5  "4"
  P*/1 -> Pos*/7  "6"
  Pos*/1 -> PosError/1, Pos/1
  Current2Volt/1 -> CurrentVolt/1  "Votl (-+10V)"

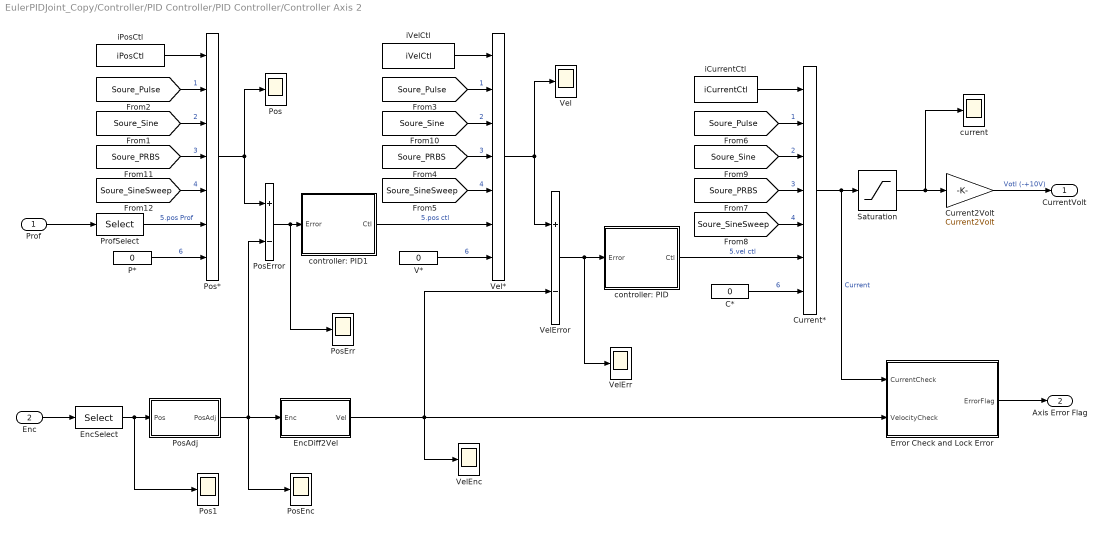
== system EulerPIDJoint_Copy/Controller/PID Controller/PID Controller/Controller Axis 2 ==
  Prof : Inport
  Enc : Inport  Port=2
  C* : Constant  Value=0  SampleTime=Ts
  Current* : MultiPortSwitch  Inputs=6  zeroidx=off
  Current2Volt : Gain  Gain=Current2Volt
  EncDiff2Vel : Subsystem
  "EncSelect " : Selector  InputPortWidth=6  IndexOptions=Index vector (dialog)  Indices=AxisNO  OutputSizes=1
  Error Check and Lock Error : Subsystem
  P* : Constant  Value=0  SampleTime=Ts
  Pos : Scope
      settings: TimeRange=1.4  YMin=-1  YMax=1  SaveName=ScopeData2
  Pos* : MultiPortSwitch  Inputs=6  zeroidx=off
  Pos1 : Scope
      settings: TimeRange=10  YMin=-1  YMax=1  SaveName=ScopeData35
  PosAdj : Subsystem
  PosEnc : Scope
      settings: TimeRange=10  YMin=-1  YMax=1  SaveName=ScopeData39
  PosErr : Scope
      settings: TimeRange=10  YMin=-1  YMax=1  SaveName=ScopeData34
  PosError : Sum  Inputs=+-
  ProfSelect : Selector  InputPortWidth=6  IndexOptions=Index vector (dialog)  Indices=AxisNO  OutputSizes=1
  Saturation : Saturate  UpperLimit=VLLimit %A  LowerLimit=-VLLimit %A  SampleTime=Ts
      settings: AttributesFormatString=%<UpperLimit>\n%<LowerLimit>
  V* : Constant  Value=0  SampleTime=Ts
  Vel : Scope
      settings: TimeRange=10  YMin=-1  YMax=1  SaveName=ScopeData5
  Vel* : MultiPortSwitch  Inputs=6  zeroidx=off
  VelEnc : Scope
      settings: TimeRange=10  YMin=-1  YMax=1  SaveName=ScopeData40
  VelErr : Scope
      settings: TimeRange=10  YMin=-1  YMax=1  SaveName=ScopeData41
  VelError : Sum  Inputs=+-
  controller: PID : Subsystem  mask{Kp=VLKp, Ki=VLKi, Kd=0, LimitSet=VLLimit, Ts=Ts}
      mask prompts: LimitSet "Limit of Int"; Ts "Sample Time"
  controller: PID1 : Subsystem  mask{Kp=PLKp, Ki=0, Kd=0, LimitSet=PLLimit, Ts=Ts}
      mask prompts: LimitSet "Limit of Int"; Ts "Sample Time"
  current : Scope
      settings: TimeRange=12  YMin=-9  YMax=9  SaveName=ScopeData3
  iCurrentCtl : Constant  Value=iCurrentCtl  SampleTime=Ts
  iPosCtl : Constant  Value=iPosCtl  SampleTime=Ts
  iVelCtl : Constant  Value=iVelCtl  SampleTime=Ts
  CurrentVolt : Outport
  Axis Error Flag : Outport  Port=2
  wires:
  Pos*/1 -> Pos/1, PosError/1
  P*/1 -> Pos*/7  "6"
  [Soure_SineSweep] -> Pos*/5  "4"
  [Soure_PRBS] -> Pos*/4  "3"
  [Soure_Sine] -> Pos*/3  "2"
  [Soure_Pulse] -> Pos*/2  "1"
  ProfSelect/1 -> Pos*/6  "5.pos Prof"
  iPosCtl/1 -> Pos*/1
  Vel*/1 -> Vel/1, VelError/1
  V*/1 -> Vel*/7  "6"
  [Soure_SineSweep] -> Vel*/5  "4"
  [Soure_PRBS] -> Vel*/4  "3"
  [Soure_Sine] -> Vel*/3  "2"
  [Soure_Pulse] -> Vel*/2  "1"
  C*/1 -> Current*/7  "6"
  controller: PID/1(Ctl) -> Current*/6  "5.vel ctl"
  [Soure_SineSweep] -> Current*/5  "4"
  [Soure_PRBS] -> Current*/4  "3"
  [Soure_Sine] -> Current*/3  "2"
  [Soure_Pulse] -> Current*/2  "1"
  "EncSelect "/1 -> PosAdj/1(Pos), Pos1/1
  Enc/1 -> "EncSelect "/1
  Prof/1 -> ProfSelect/1
  EncDiff2Vel/1(Vel) -> Error Check and Lock Error/2(VelocityCheck), VelEnc/1, VelError/2
  PosAdj/1(PosAdj) -> EncDiff2Vel/1(Enc), PosEnc/1, PosError/2
  controller: PID1/1(Ctl) -> Vel*/6  "5.pos ctl"
  VelError/1 -> controller: PID/1(Error), VelErr/1
  iVelCtl/1 -> Vel*/1
  iCurrentCtl/1 -> Current*/1
  PosError/1 -> controller: PID1/1(Error), PosErr/1
  Current*/1 -> Saturation/1, Error Check and Lock Error/1(CurrentCheck)  "Current"
  Saturation/1 -> current/1, Current2Volt/1
  Current2Volt/1 -> CurrentVolt/1  "Votl (-+10V)"
  Error Check and Lock Error/1(ErrorFlag) -> Axis Error Flag/1

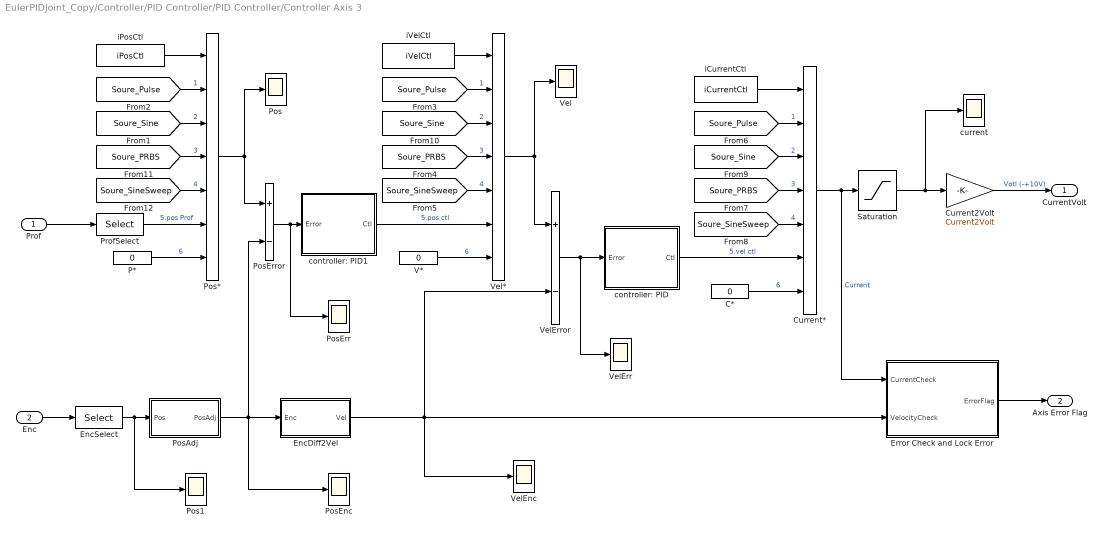
== system EulerPIDJoint_Copy/Controller/PID Controller/PID Controller/Controller Axis 3 ==
  Prof : Inport
  Enc : Inport  Port=2
  C* : Constant  Value=0  SampleTime=Ts
  Current* : MultiPortSwitch  Inputs=6  zeroidx=off
  Current2Volt : Gain  Gain=Current2Volt
  EncDiff2Vel : Subsystem
  "EncSelect " : Selector  InputPortWidth=6  IndexOptions=Index vector (dialog)  Indices=AxisNO  OutputSizes=1
  Error Check and Lock Error : Subsystem
  P* : Constant  Value=0  SampleTime=Ts
  Pos : Scope
      settings: TimeRange=1.4  YMin=-1  YMax=1  SaveName=ScopeData2
  Pos* : MultiPortSwitch  Inputs=6  zeroidx=off
  Pos1 : Scope
      settings: TimeRange=10  YMin=-1  YMax=1  SaveName=ScopeData20
  PosAdj : Subsystem
  PosEnc : Scope
      settings: TimeRange=10  YMin=-1  YMax=1  SaveName=ScopeData21
  PosErr : Scope
      settings: TimeRange=10  YMin=-1  YMax=1  SaveName=ScopeData22
  PosError : Sum  Inputs=+-
  ProfSelect : Selector  InputPortWidth=6  IndexOptions=Index vector (dialog)  Indices=AxisNO  OutputSizes=1
  Saturation : Saturate  UpperLimit=VLLimit %A  LowerLimit=-VLLimit %A  SampleTime=Ts
      settings: AttributesFormatString=%<UpperLimit>\n%<LowerLimit>
  V* : Constant  Value=0  SampleTime=Ts
  Vel : Scope
      settings: TimeRange=10  YMin=-1  YMax=1  SaveName=ScopeData5
  Vel* : MultiPortSwitch  Inputs=6  zeroidx=off
  VelEnc : Scope
      settings: TimeRange=10  YMin=-1  YMax=1  SaveName=ScopeData24
  VelErr : Scope
      settings: TimeRange=10  YMin=-1  YMax=1  SaveName=ScopeData23
  VelError : Sum  Inputs=+-
  controller: PID : Subsystem  mask{Kp=VLKp, Ki=VLKi, Kd=0, LimitSet=VLLimit, Ts=Ts}
      mask prompts: LimitSet "Limit of Int"; Ts "Sample Time"
  controller: PID1 : Subsystem  mask{Kp=PLKp, Ki=0, Kd=0, LimitSet=PLLimit, Ts=Ts}
      mask prompts: LimitSet "Limit of Int"; Ts "Sample Time"
  current : Scope
      settings: TimeRange=12  YMin=-9  YMax=9  SaveName=ScopeData3
  iCurrentCtl : Constant  Value=iCurrentCtl  SampleTime=Ts
  iPosCtl : Constant  Value=iPosCtl  SampleTime=Ts
  iVelCtl : Constant  Value=iVelCtl  SampleTime=Ts
  CurrentVolt : Outport
  Axis Error Flag : Outport  Port=2
  wires:
  Error Check and Lock Error/1(ErrorFlag) -> Axis Error Flag/1
  Current2Volt/1 -> CurrentVolt/1  "Votl (-+10V)"
  Saturation/1 -> Current2Volt/1, current/1
  Current*/1 -> Error Check and Lock Error/1(CurrentCheck), Saturation/1  "Current"
  PosError/1 -> controller: PID1/1(Error), PosErr/1
  iCurrentCtl/1 -> Current*/1
  iVelCtl/1 -> Vel*/1
  VelError/1 -> controller: PID/1(Error), VelErr/1
  controller: PID1/1(Ctl) -> Vel*/6  "5.pos ctl"
  PosAdj/1(PosAdj) -> EncDiff2Vel/1(Enc), PosEnc/1, PosError/2
  EncDiff2Vel/1(Vel) -> Error Check and Lock Error/2(VelocityCheck), VelEnc/1, VelError/2
  Prof/1 -> ProfSelect/1
  Enc/1 -> "EncSelect "/1
  "EncSelect "/1 -> PosAdj/1(Pos), Pos1/1
  [Soure_Pulse] -> Current*/2  "1"
  [Soure_Sine] -> Current*/3  "2"
  [Soure_PRBS] -> Current*/4  "3"
  [Soure_SineSweep] -> Current*/5  "4"
  controller: PID/1(Ctl) -> Current*/6  "5.vel ctl"
  C*/1 -> Current*/7  "6"
  [Soure_Pulse] -> Vel*/2  "1"
  [Soure_Sine] -> Vel*/3  "2"
  [Soure_PRBS] -> Vel*/4  "3"
  [Soure_SineSweep] -> Vel*/5  "4"
  V*/1 -> Vel*/7  "6"
  Vel*/1 -> VelError/1, Vel/1
  iPosCtl/1 -> Pos*/1
  ProfSelect/1 -> Pos*/6  "5.pos Prof"
  [Soure_Pulse] -> Pos*/2  "1"
  [Soure_Sine] -> Pos*/3  "2"
  [Soure_PRBS] -> Pos*/4  "3"
  [Soure_SineSweep] -> Pos*/5  "4"
  P*/1 -> Pos*/7  "6"
  Pos*/1 -> PosError/1, Pos/1

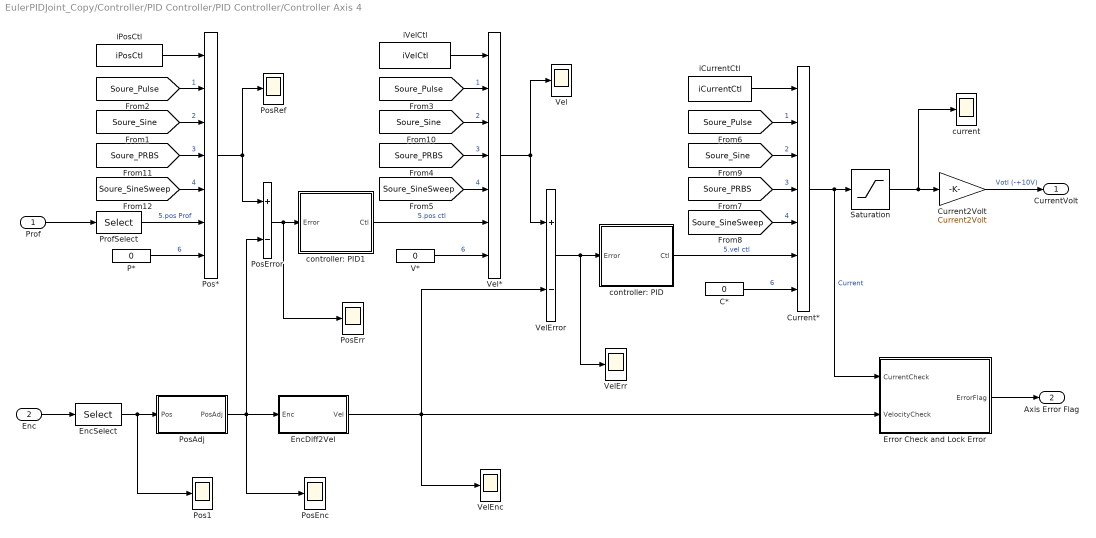
== system EulerPIDJoint_Copy/Controller/PID Controller/PID Controller/Controller Axis 4 ==
  Prof : Inport
  Enc : Inport  Port=2
  C* : Constant  Value=0  SampleTime=Ts
  Current* : MultiPortSwitch  Inputs=6  zeroidx=off
  Current2Volt : Gain  Gain=Current2Volt
  EncDiff2Vel : Subsystem
  "EncSelect " : Selector  InputPortWidth=6  IndexOptions=Index vector (dialog)  Indices=AxisNO  OutputSizes=1
  Error Check and Lock Error : Subsystem
  P* : Constant  Value=0  SampleTime=Ts
  Pos* : MultiPortSwitch  Inputs=6  zeroidx=off
  Pos1 : Scope
      settings: TimeRange=10  YMin=-1  YMax=1  SaveName=ScopeData26
  PosAdj : Subsystem
  PosEnc : Scope
      settings: TimeRange=10  YMin=-1  YMax=1  SaveName=ScopeData27
  PosErr : Scope
      settings: TimeRange=10  YMin=-1  YMax=1  SaveName=ScopeData25
  PosError : Sum  Inputs=+-
  PosRef : Scope
      settings: TimeRange=1.4  YMin=-1  YMax=1  SaveName=ScopeData2
  ProfSelect : Selector  InputPortWidth=6  IndexOptions=Index vector (dialog)  Indices=AxisNO  OutputSizes=1
  Saturation : Saturate  UpperLimit=VLLimit %A  LowerLimit=-VLLimit %A  SampleTime=Ts
      settings: AttributesFormatString=%<UpperLimit>\n%<LowerLimit>
  V* : Constant  Value=0  SampleTime=Ts
  Vel : Scope
      settings: TimeRange=10  YMin=-1  YMax=1  SaveName=ScopeData5
  Vel* : MultiPortSwitch  Inputs=6  zeroidx=off
  VelEnc : Scope
      settings: TimeRange=10  YMin=-1  YMax=1  SaveName=ScopeData29
  VelErr : Scope
      settings: TimeRange=10  YMin=-1  YMax=1  SaveName=ScopeData28
  VelError : Sum  Inputs=+-
  controller: PID : Subsystem  mask{Kp=VLKp, Ki=VLKi, Kd=0, LimitSet=VLLimit, Ts=Ts}
      mask prompts: LimitSet "Limit of Int"; Ts "Sample Time"
  controller: PID1 : Subsystem  mask{Kp=PLKp, Ki=0, Kd=0, LimitSet=PLLimit, Ts=Ts}
      mask prompts: LimitSet "Limit of Int"; Ts "Sample Time"
  current : Scope
      settings: TimeRange=12  YMin=-9  YMax=9  SaveName=ScopeData3
  iCurrentCtl : Constant  Value=iCurrentCtl  SampleTime=Ts
  iPosCtl : Constant  Value=iPosCtl  SampleTime=Ts
  iVelCtl : Constant  Value=iVelCtl  SampleTime=Ts
  CurrentVolt : Outport
  Axis Error Flag : Outport  Port=2
  wires:
  Pos*/1 -> PosRef/1, PosError/1
  P*/1 -> Pos*/7  "6"
  [Soure_SineSweep] -> Pos*/5  "4"
  [Soure_PRBS] -> Pos*/4  "3"
  [Soure_Sine] -> Pos*/3  "2"
  [Soure_Pulse] -> Pos*/2  "1"
  ProfSelect/1 -> Pos*/6  "5.pos Prof"
  iPosCtl/1 -> Pos*/1
  Vel*/1 -> Vel/1, VelError/1
  V*/1 -> Vel*/7  "6"
  [Soure_SineSweep] -> Vel*/5  "4"
  [Soure_PRBS] -> Vel*/4  "3"
  [Soure_Sine] -> Vel*/3  "2"
  [Soure_Pulse] -> Vel*/2  "1"
  C*/1 -> Current*/7  "6"
  controller: PID/1(Ctl) -> Current*/6  "5.vel ctl"
  [Soure_SineSweep] -> Current*/5  "4"
  [Soure_PRBS] -> Current*/4  "3"
  [Soure_Sine] -> Current*/3  "2"
  [Soure_Pulse] -> Current*/2  "1"
  "EncSelect "/1 -> PosAdj/1(Pos), Pos1/1
  Enc/1 -> "EncSelect "/1
  Prof/1 -> ProfSelect/1
  EncDiff2Vel/1(Vel) -> Error Check and Lock Error/2(VelocityCheck), VelEnc/1, VelError/2
  PosAdj/1(PosAdj) -> EncDiff2Vel/1(Enc), PosEnc/1, PosError/2
  controller: PID1/1(Ctl) -> Vel*/6  "5.pos ctl"
  VelError/1 -> controller: PID/1(Error), VelErr/1
  iVelCtl/1 -> Vel*/1
  iCurrentCtl/1 -> Current*/1
  PosError/1 -> controller: PID1/1(Error), PosErr/1
  Current*/1 -> Saturation/1, Error Check and Lock Error/1(CurrentCheck)  "Current"
  Saturation/1 -> current/1, Current2Volt/1
  Current2Volt/1 -> CurrentVolt/1  "Votl (-+10V)"
  Error Check and Lock Error/1(ErrorFlag) -> Axis Error Flag/1

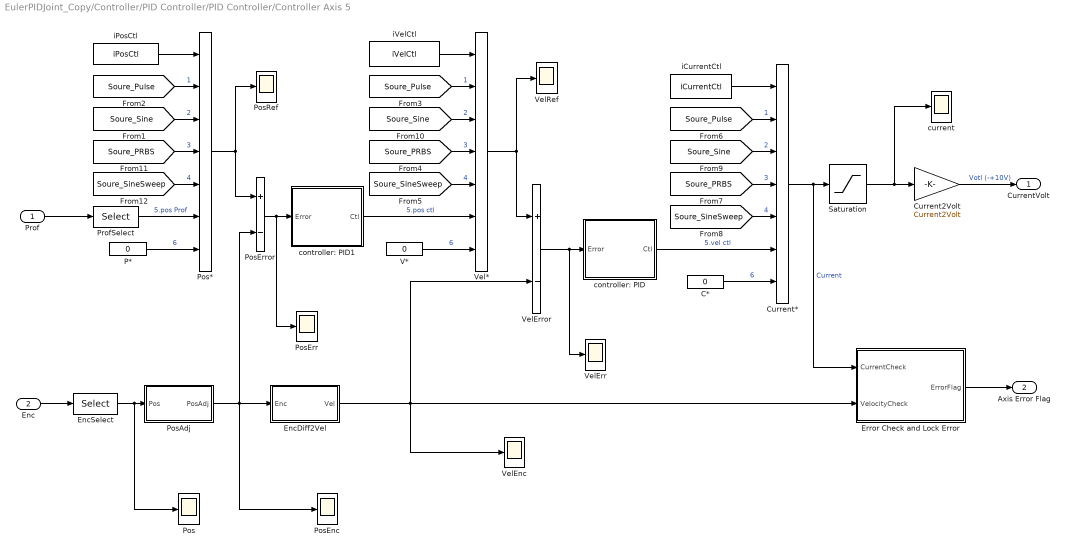
== system EulerPIDJoint_Copy/Controller/PID Controller/PID Controller/Controller Axis 5 ==
  Prof : Inport
  Enc : Inport  Port=2
  C* : Constant  Value=0  SampleTime=Ts
  Current* : MultiPortSwitch  Inputs=6  zeroidx=off
  Current2Volt : Gain  Gain=Current2Volt
  EncDiff2Vel : Subsystem
  "EncSelect " : Selector  InputPortWidth=6  IndexOptions=Index vector (dialog)  Indices=AxisNO  OutputSizes=1
  Error Check and Lock Error : Subsystem
  P* : Constant  Value=0  SampleTime=Ts
  Pos : Scope
      settings: TimeRange=10  YMin=-1  YMax=1  SaveName=ScopeData15
  Pos* : MultiPortSwitch  Inputs=6  zeroidx=off
  PosAdj : Subsystem
  PosEnc : Scope
      settings: TimeRange=10  YMin=-1  YMax=1  SaveName=ScopeData16
  PosErr : Scope
      settings: TimeRange=10  YMin=-1  YMax=1  SaveName=ScopeData19
  PosError : Sum  Inputs=+-
  PosRef : Scope
      settings: TimeRange=1.4  YMin=-1  YMax=1  SaveName=ScopeData2
  ProfSelect : Selector  InputPortWidth=6  IndexOptions=Index vector (dialog)  Indices=AxisNO  OutputSizes=1
  Saturation : Saturate  UpperLimit=VLLimit %A  LowerLimit=-VLLimit %A  SampleTime=Ts
      settings: AttributesFormatString=%<UpperLimit>\n%<LowerLimit>
  V* : Constant  Value=0  SampleTime=Ts
  Vel* : MultiPortSwitch  Inputs=6  zeroidx=off
  VelEnc : Scope
      settings: TimeRange=10  YMin=-1  YMax=1  SaveName=ScopeData17
  VelErr : Scope
      settings: TimeRange=10  YMin=-1  YMax=1  SaveName=ScopeData18
  VelError : Sum  Inputs=+-
  VelRef : Scope
      settings: TimeRange=10  YMin=-1  YMax=1  SaveName=ScopeData5
  controller: PID : Subsystem  mask{Kp=VLKp, Ki=VLKi, Kd=0, LimitSet=VLLimit, Ts=Ts}
      mask prompts: LimitSet "Limit of Int"; Ts "Sample Time"
  controller: PID1 : Subsystem  mask{Kp=PLKp, Ki=0, Kd=0, LimitSet=PLLimit, Ts=Ts}
      mask prompts: LimitSet "Limit of Int"; Ts "Sample Time"
  current : Scope
      settings: TimeRange=12  YMin=-9  YMax=9  SaveName=ScopeData3
  iCurrentCtl : Constant  Value=iCurrentCtl  SampleTime=Ts
  iPosCtl : Constant  Value=iPosCtl  SampleTime=Ts
  iVelCtl : Constant  Value=iVelCtl  SampleTime=Ts
  CurrentVolt : Outport
  Axis Error Flag : Outport  Port=2
  wires:
  Error Check and Lock Error/1(ErrorFlag) -> Axis Error Flag/1
  Current2Volt/1 -> CurrentVolt/1  "Votl (-+10V)"
  Saturation/1 -> Current2Volt/1, current/1
  Current*/1 -> Error Check and Lock Error/1(CurrentCheck), Saturation/1  "Current"
  PosError/1 -> controller: PID1/1(Error), PosErr/1
  iCurrentCtl/1 -> Current*/1
  iVelCtl/1 -> Vel*/1
  VelError/1 -> controller: PID/1(Error), VelErr/1
  controller: PID1/1(Ctl) -> Vel*/6  "5.pos ctl"
  PosAdj/1(PosAdj) -> EncDiff2Vel/1(Enc), PosEnc/1, PosError/2
  EncDiff2Vel/1(Vel) -> Error Check and Lock Error/2(VelocityCheck), VelEnc/1, VelError/2
  Prof/1 -> ProfSelect/1
  Enc/1 -> "EncSelect "/1
  "EncSelect "/1 -> PosAdj/1(Pos), Pos/1
  [Soure_Pulse] -> Current*/2  "1"
  [Soure_Sine] -> Current*/3  "2"
  [Soure_PRBS] -> Current*/4  "3"
  [Soure_SineSweep] -> Current*/5  "4"
  controller: PID/1(Ctl) -> Current*/6  "5.vel ctl"
  C*/1 -> Current*/7  "6"
  [Soure_Pulse] -> Vel*/2  "1"
  [Soure_Sine] -> Vel*/3  "2"
  [Soure_PRBS] -> Vel*/4  "3"
  [Soure_SineSweep] -> Vel*/5  "4"
  V*/1 -> Vel*/7  "6"
  Vel*/1 -> VelRef/1, VelError/1
  iPosCtl/1 -> Pos*/1
  ProfSelect/1 -> Pos*/6  "5.pos Prof"
  [Soure_Pulse] -> Pos*/2  "1"
  [Soure_Sine] -> Pos*/3  "2"
  [Soure_PRBS] -> Pos*/4  "3"
  [Soure_SineSweep] -> Pos*/5  "4"
  P*/1 -> Pos*/7  "6"
  Pos*/1 -> PosError/1, PosRef/1

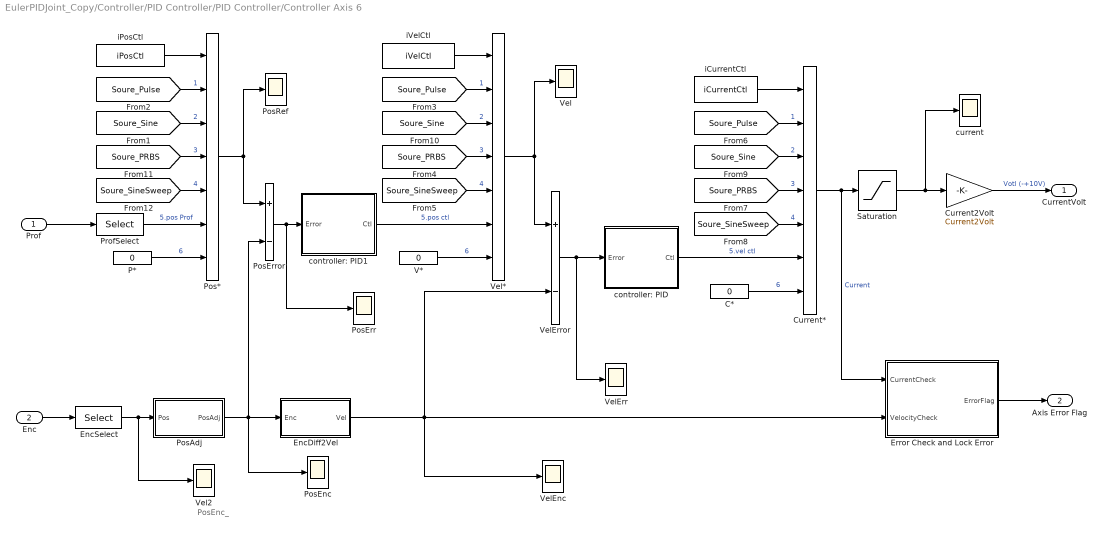
== system EulerPIDJoint_Copy/Controller/PID Controller/PID Controller/Controller Axis 6 ==
  note: PosEnc_
  Prof : Inport
  Enc : Inport  Port=2
  C* : Constant  Value=0  SampleTime=Ts
  Current* : MultiPortSwitch  Inputs=6  zeroidx=off
  Current2Volt : Gain  Gain=Current2Volt
  EncDiff2Vel : Subsystem
  "EncSelect " : Selector  InputPortWidth=6  IndexOptions=Index vector (dialog)  Indices=AxisNO  OutputSizes=1
  Error Check and Lock Error : Subsystem
  P* : Constant  Value=0  SampleTime=Ts
  Pos* : MultiPortSwitch  Inputs=6  zeroidx=off
  PosAdj : Subsystem
  PosEnc : Scope
      settings: TimeRange=10  YMin=-1  YMax=1  SaveName=ScopeData14
  PosErr : Scope
      settings: TimeRange=10  YMin=-1  YMax=1  SaveName=ScopeData12
  PosError : Sum  Inputs=+-
  PosRef : Scope
      settings: TimeRange=1.4  YMin=-1  YMax=1  SaveName=ScopeData2
  ProfSelect : Selector  InputPortWidth=6  IndexOptions=Index vector (dialog)  Indices=AxisNO  OutputSizes=1
  Saturation : Saturate  UpperLimit=VLLimit %A  LowerLimit=-VLLimit %A  SampleTime=Ts
      settings: AttributesFormatString=%<UpperLimit>\n%<LowerLimit>
  V* : Constant  Value=0  SampleTime=Ts
  Vel : Scope
      settings: TimeRange=10  YMin=-1  YMax=1  SaveName=ScopeData5
  Vel* : MultiPortSwitch  Inputs=6  zeroidx=off
  Vel2 : Scope
      settings: TimeRange=10  YMin=-1  YMax=1  SaveName=ScopeData13
  VelEnc : Scope
      settings: TimeRange=10  YMin=-1  YMax=1  SaveName=ScopeData48
  VelErr : Scope
      settings: TimeRange=10  YMin=-1  YMax=1  SaveName=ScopeData47
  VelError : Sum  Inputs=+-
  controller: PID : Subsystem  mask{Kp=VLKp, Ki=VLKi, Kd=0, LimitSet=VLLimit, Ts=Ts}
      mask prompts: LimitSet "Limit of Int"; Ts "Sample Time"
  controller: PID1 : Subsystem  mask{Kp=PLKp, Ki=0, Kd=0, LimitSet=PLLimit, Ts=Ts}
      mask prompts: LimitSet "Limit of Int"; Ts "Sample Time"
  current : Scope
      settings: TimeRange=12  YMin=-9  YMax=9  SaveName=ScopeData3
  iCurrentCtl : Constant  Value=iCurrentCtl  SampleTime=Ts
  iPosCtl : Constant  Value=iPosCtl  SampleTime=Ts
  iVelCtl : Constant  Value=iVelCtl  SampleTime=Ts
  CurrentVolt : Outport
  Axis Error Flag : Outport  Port=2
  wires:
  Pos*/1 -> PosRef/1, PosError/1
  P*/1 -> Pos*/7  "6"
  [Soure_SineSweep] -> Pos*/5  "4"
  [Soure_PRBS] -> Pos*/4  "3"
  [Soure_Sine] -> Pos*/3  "2"
  [Soure_Pulse] -> Pos*/2  "1"
  ProfSelect/1 -> Pos*/6  "5.pos Prof"
  iPosCtl/1 -> Pos*/1
  Vel*/1 -> Vel/1, VelError/1
  V*/1 -> Vel*/7  "6"
  [Soure_SineSweep] -> Vel*/5  "4"
  [Soure_PRBS] -> Vel*/4  "3"
  [Soure_Sine] -> Vel*/3  "2"
  [Soure_Pulse] -> Vel*/2  "1"
  C*/1 -> Current*/7  "6"
  controller: PID/1(Ctl) -> Current*/6  "5.vel ctl"
  [Soure_SineSweep] -> Current*/5  "4"
  [Soure_PRBS] -> Current*/4  "3"
  [Soure_Sine] -> Current*/3  "2"
  [Soure_Pulse] -> Current*/2  "1"
  "EncSelect "/1 -> PosAdj/1(Pos), Vel2/1
  Enc/1 -> "EncSelect "/1
  Prof/1 -> ProfSelect/1
  EncDiff2Vel/1(Vel) -> Error Check and Lock Error/2(VelocityCheck), VelEnc/1, VelError/2
  PosAdj/1(PosAdj) -> EncDiff2Vel/1(Enc), PosEnc/1, PosError/2
  controller: PID1/1(Ctl) -> Vel*/6  "5.pos ctl"
  VelError/1 -> controller: PID/1(Error), VelErr/1
  iVelCtl/1 -> Vel*/1
  iCurrentCtl/1 -> Current*/1
  PosError/1 -> controller: PID1/1(Error), PosErr/1
  Current*/1 -> Saturation/1, Error Check and Lock Error/1(CurrentCheck)  "Current"
  Saturation/1 -> current/1, Current2Volt/1
  Current2Volt/1 -> CurrentVolt/1  "Votl (-+10V)"
  Error Check and Lock Error/1(ErrorFlag) -> Axis Error Flag/1

== system EulerPIDJoint_Copy/Controller/PID Controller/PID Controller/Source Model ==
  EncDiff2Vel : Subsystem
  PRBS_Offset : Constant  Value=PRBSOffset  SampleTime=Ts
  Product : Product  RndMeth=Zero
  Pulse : ToWorkspace  VariableName=RefPulse  SampleTime=-1  SaveFormat=Structure
  Vel1 : Scope
      settings: TimeRange=4.5  YMin=-50  YMax=50  SaveName=ScopeData8
  Vel2 : Scope
      settings: TimeRange=4.5  YMin=-50  YMax=50  SaveName=ScopeData4
  add : Sum
  b.Source_Ctl : Constant  SampleTime=Ts
  b.Source_PRBS_Offset : Constant  Value=0  SampleTime=Ts
  source: PRBS : Subsystem  mask{CurrentValue=PRBSGain, BandStop=1/4    %2kHz, TL=PRBSTimeLength, Ts=Ts}
      mask prompts: CurrentValue "The Value of Current"; BandStop "band stop parameter: 1 for 32KHz"; TL "Time Length"; Ts "Sampe Time"
      mask init:
      | %prbs_u = idinput(TL/Ts,'prbs',[0 BandStop],[-1 1]);
      | prbs_u = idinput(TL/Ts,'prbs',[0 BandStop],[-1 1]);
  source: Pulse : Subsystem  mask{VelGain=PulseGain, Frq=PulseFrq, Ts=Ts}
      mask prompts: VelGain "Velocity Gain"; Frq "Frequence Hz"; Ts "Sample Time"
  source: SineSwp : Subsystem  mask{CurrentValue=0, BandStop=1/16 %2KHz, TL=2, Ts=Ts}
      mask prompts: CurrentValue "The Value of Current"; BandStop "band stop parameter: 1 for 32KHz"; TL "Time Length"; Ts "Sampe Time"
  source: Single : Subsystem  mask{VelGain=SineGain, Frq=SineFrq, Ts=Ts}
      mask prompts: VelGain "Velocity Gain"; Frq "Frequence Hz"; Ts "Sample Time"
  tag scope: Soure_PRBS=global, Soure_Pulse=global, Soure_Sine=global, Soure_SineSweep=global
  wires:
  source: PRBS/1(PRBS*) -> add/1
  Product/1 -> add/2
  PRBS_Offset/1 -> Product/2
  b.Source_PRBS_Offset/1 -> Product/1
  b.Source_Ctl/1 -> source: Single/Enable, source: SineSwp/Enable, source: Pulse/Enable, source: PRBS/Enable
  source: Single/1(Sine) -> [Soure_Sine]
  source: SineSwp/1(SineOut) -> [Soure_SineSweep]
  source: Pulse/1(Pulse) -> [Soure_Pulse], Vel1/1, EncDiff2Vel/1(Enc), Pulse/1
  add/1 -> [Soure_PRBS]
  EncDiff2Vel/1(Vel) -> Vel2/1

== system EulerPIDJoint_Copy/Display/GeneralAccDisplay/Jnt1/Display ==
  GeneralAcc1 : Inport
  Ref_GeneralAcc1 : Inport  Port=2
  AVx : Scope  NumInputPorts=2
      settings: TimeRange=10  YMin=-2.999999999999999e-017~-1  YMax=4e-017~1
  "AVy " : Scope  NumInputPorts=2
      settings: YMin=-5~-5  YMax=5~5
  AVz : Scope  NumInputPorts=2
      settings: YMin=-5~-5  YMax=5~5  SaveName=ScopeData2
  AWx : Scope  NumInputPorts=2
      settings: YMin=-5~-5  YMax=5~5  SaveName=ScopeData3
  AWy : Scope  NumInputPorts=2
      settings: TimeRange=10  YMin=-4.18~4.060000000000001  YMax=-4.04~4.2  SaveName=ScopeData4
  AWz : Scope  NumInputPorts=2
      settings: TimeRange=10  YMin=-1.6e-006~-0.003  YMax=4e-007~0.004  SaveName=ScopeData5
  Demux : Demux  Outputs=6
  Demux1 : Demux  Outputs=6
  "Encoder " : ToWorkspace  VariableName=EncGenAccJ1  SampleTime=-1  SaveFormat=Structure
  Err{1..6} (6 alike) : Scope
      Err1 settings: SaveName=ScopeData6
      Err2 settings: SaveName=ScopeData7
      Err3 settings: SaveName=ScopeData8
      Err4 settings: SaveName=ScopeData9
      Err5 settings: TimeRange=3  YMin=-2.5  YMax=1  SaveName=ScopeData10
      Err6 settings: SaveName=ScopeData11
  "Ref " : ToWorkspace  VariableName=RefGenAccJ1  SampleTime=-1  SaveFormat=Structure
  Sum{,1..5} (6 alike) : Sum  Inputs=+|-
  wires:
  Demux1/6 -> Sum5/2, AWz/2
  Demux1/5 -> Sum4/2, AWy/2
  Demux1/4 -> AWx/2, Sum3/2
  Demux1/3 -> Sum2/2, AVz/2
  Demux1/2 -> Sum1/2, "AVy "/2
  Demux/6 -> Sum5/1, AWz/1
  Demux/5 -> Sum4/1, AWy/1
  Demux/4 -> AWx/1, Sum3/1
  Demux/3 -> Sum2/1, AVz/1
  Demux/2 -> Sum1/1, "AVy "/1
  Demux1/1 -> AVx/2, Sum/2
  Demux/1 -> AVx/1, Sum/1
  Ref_GeneralAcc1/1 -> "Ref "/1, Demux1/1
  GeneralAcc1/1 -> "Encoder "/1, Demux/1
  Sum5/1 -> Err6/1
  Sum4/1 -> Err5/1
  Sum3/1 -> Err4/1
  Sum2/1 -> Err3/1
  Sum1/1 -> Err2/1
  Sum/1 -> Err1/1

== system EulerPIDJoint_Copy/Display/GeneralAccDisplay/Jnt2/Display ==
  GeneralAcc2 : Inport
  Ref_GeneralAcc2 : Inport  Port=2
  AVx : Scope  NumInputPorts=2
      settings: TimeRange=10  YMin=-2.999999999999999e-017~-1  YMax=4e-017~1
  "AVy " : Scope  NumInputPorts=2
      settings: YMin=-5~-5  YMax=5~5
  AVz : Scope  NumInputPorts=2
      settings: YMin=-5~-5  YMax=5~5  SaveName=ScopeData2
  AWx : Scope  NumInputPorts=2
      settings: YMin=-5~-5  YMax=5~5  SaveName=ScopeData3
  AWy : Scope  NumInputPorts=2
      settings: TimeRange=10  YMin=-4.18~4.060000000000001  YMax=-4.04~4.2  SaveName=ScopeData4
  AWz : Scope  NumInputPorts=2
      settings: TimeRange=10  YMin=-1.6e-006~-0.003  YMax=4e-007~0.004  SaveName=ScopeData5
  Demux : Demux  Outputs=6
  Demux1 : Demux  Outputs=6
  "Encoder " : ToWorkspace  VariableName=EncGenAccJ2  SampleTime=-1  SaveFormat=Structure
  Err{1..6} (6 alike) : Scope
      Err1 settings: SaveName=ScopeData6
      Err2 settings: SaveName=ScopeData7
      Err3 settings: SaveName=ScopeData8
      Err4 settings: SaveName=ScopeData9
      Err5 settings: TimeRange=3  YMin=-2.5  YMax=1  SaveName=ScopeData10
      Err6 settings: SaveName=ScopeData11
  "Ref " : ToWorkspace  VariableName=RefGenAccJ2  SampleTime=-1  SaveFormat=Structure
  Sum{,1..5} (6 alike) : Sum  Inputs=+|-
  wires:
  Sum/1 -> Err1/1
  Sum1/1 -> Err2/1
  Sum2/1 -> Err3/1
  Sum3/1 -> Err4/1
  Sum4/1 -> Err5/1
  Sum5/1 -> Err6/1
  GeneralAcc2/1 -> Demux/1, "Encoder "/1
  Ref_GeneralAcc2/1 -> Demux1/1, "Ref "/1
  Demux/1 -> Sum/1, AVx/1
  Demux1/1 -> Sum/2, AVx/2
  Demux/2 -> "AVy "/1, Sum1/1
  Demux/3 -> AVz/1, Sum2/1
  Demux/4 -> Sum3/1, AWx/1
  Demux/5 -> AWy/1, Sum4/1
  Demux/6 -> AWz/1, Sum5/1
  Demux1/2 -> "AVy "/2, Sum1/2
  Demux1/3 -> AVz/2, Sum2/2
  Demux1/4 -> Sum3/2, AWx/2
  Demux1/5 -> AWy/2, Sum4/2
  Demux1/6 -> AWz/2, Sum5/2
